simulink model "Task02"  (R2015a)
settings: Solver=ode45  StartTime=0.0  StopTime=10.0  RelTol=1e-3
libraries: cstblocks x5, simulink x1
settings Model: Creator=Ashfaq  LastModifiedBy=Ashfaq

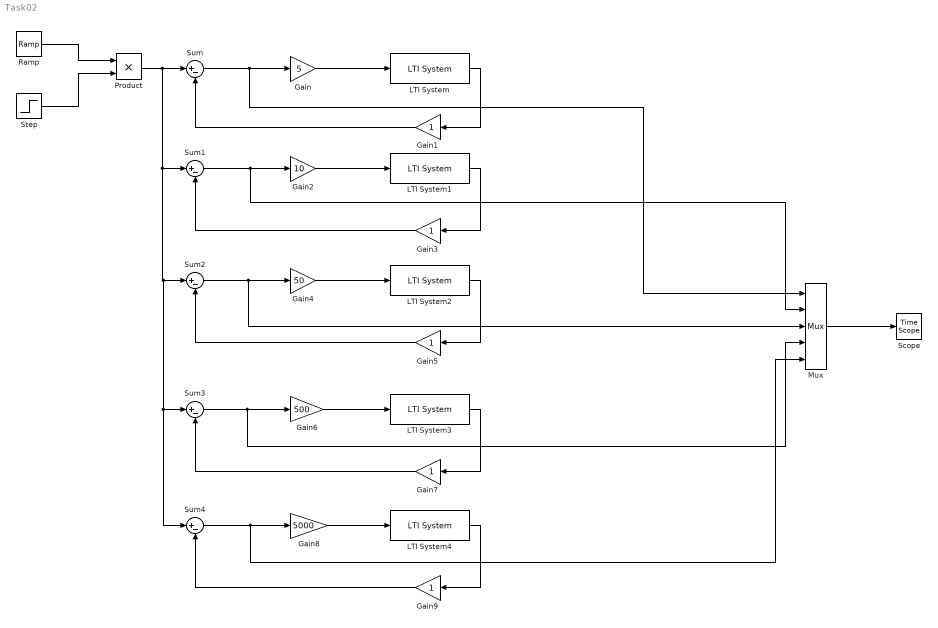
== system Task02 ==
  Gain : Gain  Gain=5
  Gain{1,3,5,7,9} (5 alike) : Gain
  Gain2 : Gain  Gain=10
  Gain4 : Gain  Gain=50
  Gain6 : Gain  Gain=500
  Gain8 : Gain  Gain=5000
  LTI System{,1..4} (5 alike) : cstblocks/LTI System  sys=tf([1 6],[1 32 367 1776 3024])  IC=[]
  Mux : Mux  Inputs=5
  Product : Product
  Ramp : simulink/Sources/Ramp  slope=1  start=0  X0=0
  Scope : TimeScope
  Step : Step  After=5  SampleTime=0
  Sum{,1..4} (5 alike) : Sum  Inputs=|+-
  wires:
  Sum/1 -> Mux/1, Gain/1
  Gain/1 -> LTI System/1
  LTI System/1 -> Gain1/1
  Gain1/1 -> Sum/2
  Sum1/1 -> Mux/2, Gain2/1
  Gain2/1 -> LTI System1/1
  LTI System1/1 -> Gain3/1
  Gain3/1 -> Sum1/2
  Sum2/1 -> Mux/3, Gain4/1
  Gain4/1 -> LTI System2/1
  LTI System2/1 -> Gain5/1
  Gain5/1 -> Sum2/2
  Sum3/1 -> Mux/4, Gain6/1
  Gain6/1 -> LTI System3/1
  LTI System3/1 -> Gain7/1
  Gain7/1 -> Sum3/2
  Sum4/1 -> Mux/5, Gain8/1
  Gain8/1 -> LTI System4/1
  LTI System4/1 -> Gain9/1
  Gain9/1 -> Sum4/2
  Mux/1 -> Scope/1
  Product/1 -> Sum4/1, Sum3/1, Sum2/1, Sum1/1, Sum/1
  Step/1 -> Product/2
  Ramp/1 -> Product/1
